simulink subsystem "TurbinePitchControllerSubsystem"  (R2023b)
settings: Solver=VariableStepAuto  StartTime=0.0  StopTime=10.0  RelTol=1e-3
values from neighbouring files (symbols this model uses):
  actuatorRampRate = 20    [wind_turbine_inputs.m]
  controllerTimeConstant = 2    [wind_turbine_inputs.m]
  iGenerationGain = 1    [wind_turbine_inputs.m]
  maxPitchAngle = max(pitch)    [wind_turbine_inputs.m]
  minPitchAngle = min(pitch)    [wind_turbine_inputs.m]
  pGenerationGain = 0.1    [wind_turbine_inputs.m]
  pitchBrakeAngle = 95    [wind_turbine_inputs.m]
  turbineRatedPower = 1.5    [wind_turbine_inputs.m]
undefined symbols (not defined in the file or in its folder): Derating
libraries: simulink x4
settings Model: Creator=FRESH  LastModifiedBy=FRESH

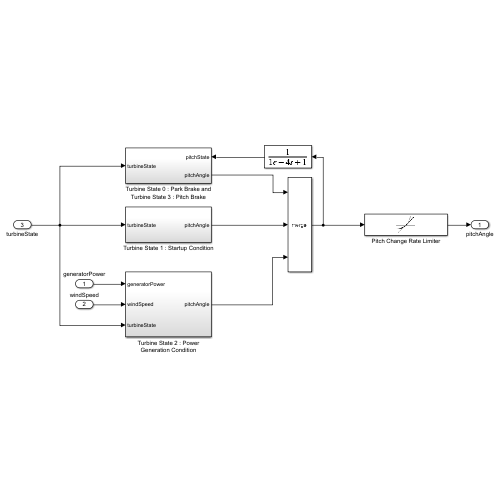
[thumbnail: Simulink's stored preview of the top-level diagram]
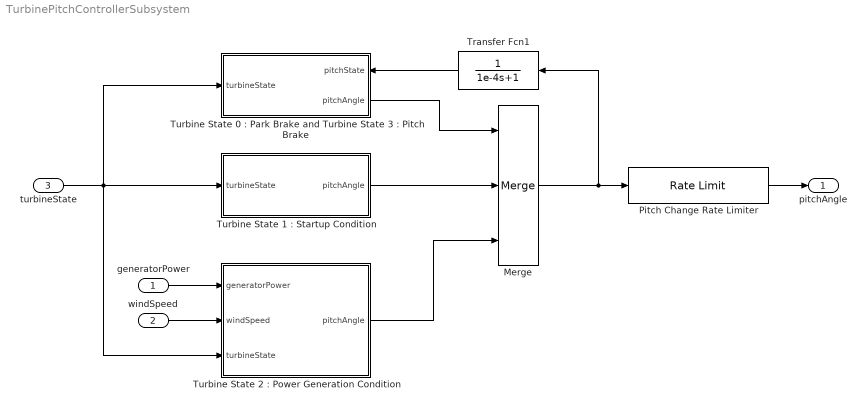
== system TurbinePitchControllerSubsystem ==
  generatorPower : Inport
  windSpeed : Inport  Port=2
  turbineState : Inport  Port=3
  Merge : Merge  Inputs=3
  Pitch Change Rate Limiter : RateLimiter  RisingSlewLimit=actuatorRampRate  FallingSlewLimit=-actuatorRampRate  SampleTimeMode=inherited
  Transfer Fcn1 : TransferFcn  Denominator=[1e-4 1]
  "Turbine State 0 : Park Brake and Turbine State 3 : Pitch Brake" : Subsystem
      settings: PortSchema="{\"entries\":[{\"content\":{\"sides\":[{\"content\":{\"connectorIds\":[\"In1\"]},\"type\":\"ConnectorPlacement.EquallySpacedRectSide\",\"uuid\":\"c81c0fc4-0b31-4a43-acf3-ef02f67f12ef\"},{\"content\":{\"connectorIds\":[\"In2\",\"Out1\"],\"side\":\"RIGHT\"},\"type\":\"ConnectorPlacement.EquallySpacedRectSide\",\"uuid\":\"c20c9bc8-a4c7-4c6f-a8fa-fe8ff88298f7\"},{\"content\":{\"connectorIds\":[],\"side\":\"TOP\"},\"type\":\"ConnectorPlacement.EquallySpacedRectSide\",\"uuid\":\"2b845051-401f-423c-a453-0a1243a015d1\"}]},\"type\":\"ConnectorPlacement.EquallySpacedConnector\",\"uuid\":\"502647d6-ee95-4637-92b5-6d3c38784edf\"}],\"packageUris\":[\"http://schema.mathworks.com/mf0/Connector/R2020b\"],\"version\":\"1.0\"}"
  "Turbine State 1 : Startup Condition" : Subsystem
  "Turbine State 2 : Power Generation Condition" : Subsystem
  pitchAngle : Outport
  wires:
  Transfer Fcn1/1 -> "Turbine State 0 : Park Brake and Turbine State 3 : Pitch Brake"/2(pitchState)
  Merge/1 -> Transfer Fcn1/1, Pitch Change Rate Limiter/1
  windSpeed/1 -> "Turbine State 2 : Power Generation Condition"/2(windSpeed)
  "Turbine State 2 : Power Generation Condition"/1(pitchAngle) -> Merge/3
  turbineState/1 -> "Turbine State 1 : Startup Condition"/1(turbineState), "Turbine State 0 : Park Brake and Turbine State 3 : Pitch Brake"/1(turbineState), "Turbine State 2 : Power Generation Condition"/3(turbineState)
  "Turbine State 1 : Startup Condition"/1(pitchAngle) -> Merge/2
  "Turbine State 0 : Park Brake and Turbine State 3 : Pitch Brake"/1(pitchAngle) -> Merge/1
  generatorPower/1 -> "Turbine State 2 : Power Generation Condition"/1(generatorPower)
  Pitch Change Rate Limiter/1 -> pitchAngle/1

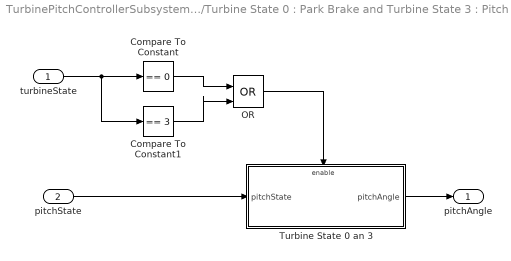
== system TurbinePitchControllerSubsystem/Turbine State 0 : Park Brake and Turbine State 3 : Pitch Brake ==
  turbineState : Inport
  pitchState : Inport  Port=2
  Compare To Constant : simulink/Logic and Bit Operations/Compare To Constant  relop===  const=0  OutDataTypeStr=boolean
  Compare To Constant1 : simulink/Logic and Bit Operations/Compare To Constant  relop===  const=3  OutDataTypeStr=boolean
  OR : Logic  Operator=OR  IconShape=distinctive  AllPortsSameDT=off  OutDataTypeStr=boolean
  Turbine State 0 an 3 : Subsystem
  pitchAngle : Outport
  wires:
  Compare To Constant1/1 -> OR/2
  Compare To Constant/1 -> OR/1
  OR/1 -> Turbine State 0 an 3/Enable
  pitchState/1 -> Turbine State 0 an 3/1(pitchState)
  turbineState/1 -> Compare To Constant/1, Compare To Constant1/1
  Turbine State 0 an 3/1(pitchAngle) -> pitchAngle/1

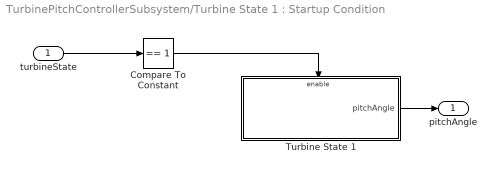
== system TurbinePitchControllerSubsystem/Turbine State 1 : Startup Condition ==
  turbineState : Inport
  Compare To Constant : simulink/Logic and Bit Operations/Compare To Constant  relop===  const=1  OutDataTypeStr=boolean
  Turbine State 1 : Subsystem
  pitchAngle : Outport
  wires:
  Turbine State 1/1(pitchAngle) -> pitchAngle/1
  Compare To Constant/1 -> Turbine State 1/Enable
  turbineState/1 -> Compare To Constant/1

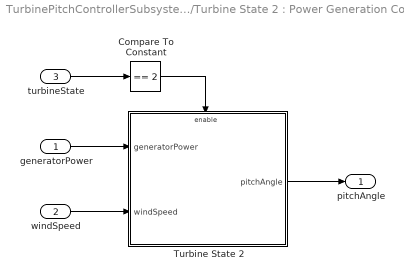
== system TurbinePitchControllerSubsystem/Turbine State 2 : Power Generation Condition ==
  generatorPower : Inport
  windSpeed : Inport  Port=2
  turbineState : Inport  Port=3
  Compare To Constant : simulink/Logic and Bit Operations/Compare To Constant  relop===  const=2  OutDataTypeStr=boolean
  Turbine State 2 : Subsystem
  pitchAngle : Outport
  wires:
  windSpeed/1 -> Turbine State 2/2(windSpeed)
  generatorPower/1 -> Turbine State 2/1(generatorPower)
  turbineState/1 -> Compare To Constant/1
  Compare To Constant/1 -> Turbine State 2/Enable
  Turbine State 2/1(pitchAngle) -> pitchAngle/1

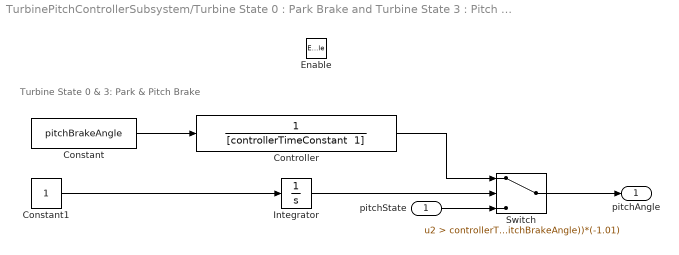
== system TurbinePitchControllerSubsystem/Turbine State 0 : Park Brake and Turbine State 3 : Pitch Brake/Turbine State 0 an 3 ==
  note: Turbine State 0 & 3: Park & Pitch Brake
  pitchState : Inport
  Enable : EnablePort  StatesWhenEnabling=reset
  Constant : Constant  Value=pitchBrakeAngle
  Constant1 : Constant
  Controller : TransferFcn  Denominator="[controllerTimeConstant  1]"
  Integrator : Integrator
  Switch : Switch  Criteria=u2 > Threshold  Threshold=controllerTimeConstant*log(1-(maxPitchAngle/pitchBrakeAngle))*(-1.01)  SaturateOnIntegerOverflow=off  InputSameDT=off
  pitchAngle : Outport
  wires:
  Switch/1 -> pitchAngle/1
  Controller/1 -> Switch/1
  Constant/1 -> Controller/1
  Constant1/1 -> Integrator/1
  pitchState/1 -> Switch/3
  Integrator/1 -> Switch/2

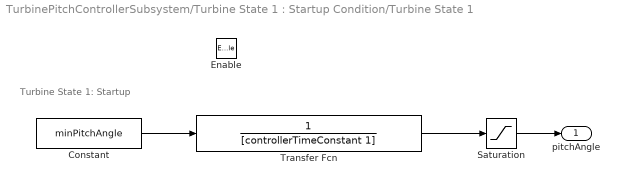
== system TurbinePitchControllerSubsystem/Turbine State 1 : Startup Condition/Turbine State 1 ==
  note: Turbine State 1: Startup
  Enable : EnablePort  StatesWhenEnabling=reset
  Constant : Constant  Value=minPitchAngle
  Saturation : Saturate  UpperLimit=maxPitchAngle  LowerLimit=minPitchAngle
  Transfer Fcn : TransferFcn  Denominator=[controllerTimeConstant 1]
  pitchAngle : Outport
  wires:
  Transfer Fcn/1 -> Saturation/1
  Saturation/1 -> pitchAngle/1
  Constant/1 -> Transfer Fcn/1

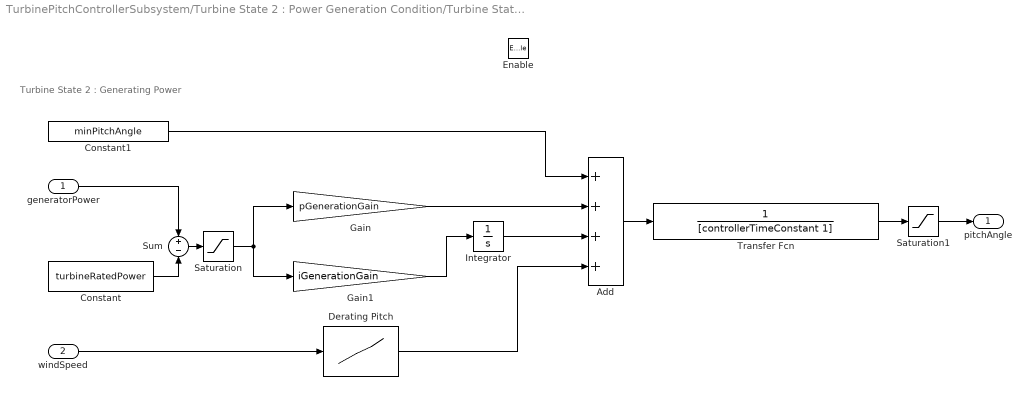
== system TurbinePitchControllerSubsystem/Turbine State 2 : Power Generation Condition/Turbine State 2 ==
  note: Turbine State 2 : Generating Power
  generatorPower : Inport
  windSpeed : Inport  Port=2
  Enable : EnablePort  StatesWhenEnabling=reset
  Add : Sum  Inputs=++++
  Constant : Constant  Value=turbineRatedPower
  Constant1 : Constant  Value=minPitchAngle
  Derating Pitch : Lookup_n-D  NumberOfTableDimensions=1  BreakpointsForDimension1=Derating(:,1)  Table=Derating(:,2)-minPitchAngle  InternalRulePriority=Speed  RndMeth=Simplest
  Gain : Gain  Gain=pGenerationGain
  Gain1 : Gain  Gain=iGenerationGain
  Integrator : Integrator
  Saturation : Saturate  UpperLimit=inf  LowerLimit=0
  Saturation1 : Saturate  UpperLimit=maxPitchAngle  LowerLimit=minPitchAngle
  Sum : Sum  Inputs=+-
  Transfer Fcn : TransferFcn  Denominator=[controllerTimeConstant 1]
  pitchAngle : Outport
  wires:
  Derating Pitch/1 -> Add/4
  windSpeed/1 -> Derating Pitch/1
  Gain1/1 -> Integrator/1
  Integrator/1 -> Add/3
  Transfer Fcn/1 -> Saturation1/1
  Saturation/1 -> Gain1/1, Gain/1
  Sum/1 -> Saturation/1
  Constant/1 -> Sum/2
  generatorPower/1 -> Sum/1
  Add/1 -> Transfer Fcn/1
  Constant1/1 -> Add/1
  Gain/1 -> Add/2
  Saturation1/1 -> pitchAngle/1
